simulink model "lab06_07_many"  (R2018b)
settings: Solver=VariableStepAuto  StartTime=0.0  StopTime=10.0  FixedStep=0.00001  RelTol=1e-3
settings Model: Creator=Еня  LastModifiedBy=Еня

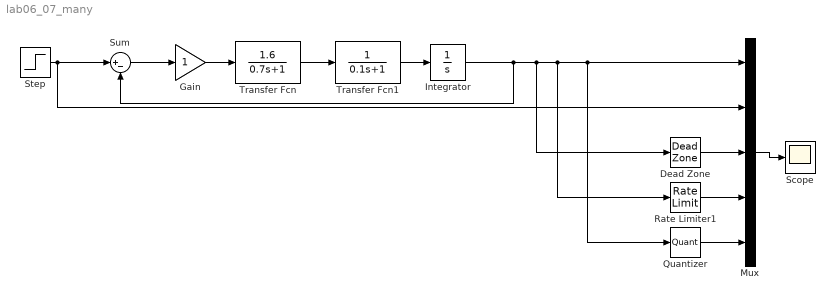
== system lab06_07_many ==
  Dead Zone : DeadZone  LowerValue=0.9  UpperValue=1.1  SaturateOnIntegerOverflow=on
  Gain : Gain
  Integrator : Integrator
  Mux : Mux  Inputs=5
  Quantizer : Quantizer
  Rate Limiter1 : RateLimiter  RisingSlewLimit=0.5  FallingSlewLimit=-0.5  SampleTimeMode=inherited
  Scope : Scope
  Step : Step  Time=0  SampleTime=0
  Sum : Sum  Inputs=|+-
  Transfer Fcn : TransferFcn  Numerator=[1.6]  Denominator=[0.7 1]
  Transfer Fcn1 : TransferFcn  Denominator=[0.1 1]
  wires:
  Step/1 -> Mux/2, Sum/1
  Sum/1 -> Gain/1
  Gain/1 -> Transfer Fcn/1
  Transfer Fcn/1 -> Transfer Fcn1/1
  Transfer Fcn1/1 -> Integrator/1
  Mux/1 -> Scope/1
  Integrator/1 -> Dead Zone/1, Rate Limiter1/1, Quantizer/1, Mux/1, Sum/2
  Dead Zone/1 -> Mux/3
  Rate Limiter1/1 -> Mux/4
  Quantizer/1 -> Mux/5
